simulink model "UnpackUDP"  (R2018b)
settings: configuration reference "Active" (kept outside this file)
undefined symbols (not defined in the file): tS, TUMHealthStatus
libraries: misc x5, etargetslib x5, simulink x2
settings Model: DataDictionary=UnpackUDP.sldd  sg_rtwmakecfg_data=_sg_IO821__sglibc_  Creator=lab1  LastModifiedBy=ge34qer

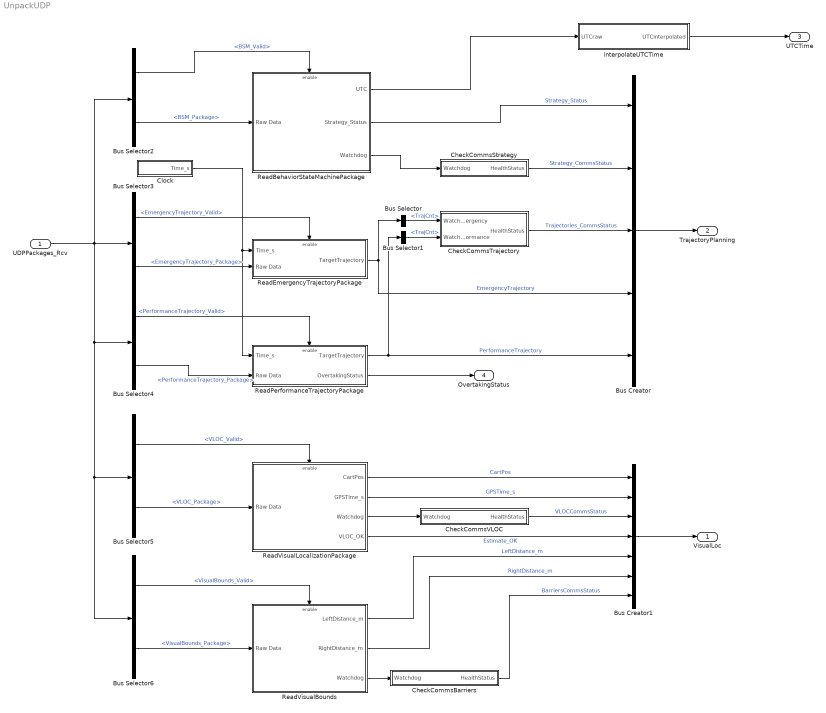
== system UnpackUDP ==
  UDPPackages_Rcv : Inport  OutDataTypeStr=Bus: UDPPackages_Rcv
  Bus Creator : BusCreator  Inputs=5
  Bus Creator1 : BusCreator  Inputs=7
  Bus Selector : BusSelector  OutputSignals=TrajCnt
  Bus Selector1 : BusSelector  OutputSignals=TrajCnt
  Bus Selector2 : BusSelector  OutputSignals=BSM_Valid,BSM_Package
  Bus Selector3 : BusSelector  OutputSignals=EmergencyTrajectory_Valid,EmergencyTrajectory_Package
  Bus Selector4 : BusSelector  OutputSignals=PerformanceTrajectory_Valid,PerformanceTrajectory_Package
  Bus Selector5 : BusSelector  OutputSignals=VLOC_Valid,VLOC_Package
  Bus Selector6 : BusSelector  OutputSignals=VisualBounds_Valid,VisualBounds_Package
  CheckCommsBarriers : Subsystem
  CheckCommsStrategy : Subsystem
  CheckCommsTrajectory : Subsystem
  CheckCommsVLOC : Subsystem
  Clock : Subsystem
  ReadBehaviorStateMachinePackage : Subsystem  Priority=1000
  ReadEmergencyTrajectoryPackage : Subsystem  Priority=1000
  ReadPerformanceTrajectoryPackage : Subsystem  Priority=1000
  ReadVisualBounds : Subsystem  Priority=1000
  ReadVisualLocalizationPackage : Subsystem  Priority=1000
  interpolateUTCTime : Subsystem
  VisualLoc : Outport  OutDataTypeStr=Bus: VisualLoc  BusOutputAsStruct=on
  TrajectoryPlanning : Outport  Port=2  OutDataTypeStr=Bus: TrajectoryPlanning  BusOutputAsStruct=on
  UTCTime : Outport  Port=3
  OvertakingStatus : Outport  Port=4  OutDataTypeStr=uint8
  wires:
  Bus Creator/1 -> TrajectoryPlanning/1
  ReadPerformanceTrajectoryPackage/1(TargetTrajectory) -> Bus Selector1/1, Bus Creator/5  "PerformanceTrajectory"
  ReadBehaviorStateMachinePackage/2(Strategy_Status) -> Bus Creator/1  "Strategy_Status"
  ReadBehaviorStateMachinePackage/3(Watchdog) -> CheckCommsStrategy/1(Watchdog)
  Bus Creator1/1 -> VisualLoc/1
  ReadVisualLocalizationPackage/2(GPSTime_s) -> Bus Creator1/2  "GPSTime_s"
  ReadVisualLocalizationPackage/1(CartPos) -> Bus Creator1/1  "CartPos"
  CheckCommsStrategy/1(HealthStatus) -> Bus Creator/2  "Strategy_CommsStatus"
  CheckCommsTrajectory/1(HealthStatus) -> Bus Creator/3  "Trajectories_CommsStatus"
  ReadEmergencyTrajectoryPackage/1(TargetTrajectory) -> Bus Creator/4, Bus Selector/1  "EmergencyTrajectory"
  Bus Selector/1 -> CheckCommsTrajectory/1(WatchdogEmergency)  "<TrajCnt>"
  Bus Selector1/1 -> CheckCommsTrajectory/2(WatchdogPerformance)  "<TrajCnt>"
  CheckCommsVLOC/1(HealthStatus) -> Bus Creator1/3  "VLOCCommsStatus"
  ReadVisualLocalizationPackage/4(VLOC_OK) -> Bus Creator1/4  "Estimate_OK"
  Clock/1(Time_s) -> ReadPerformanceTrajectoryPackage/1(Time_s), ReadEmergencyTrajectoryPackage/1(Time_s)
  UDPPackages_Rcv/1 -> Bus Selector2/1, Bus Selector6/1, Bus Selector5/1, Bus Selector4/1, Bus Selector3/1
  Bus Selector2/1 -> ReadBehaviorStateMachinePackage/Enable  "<BSM_Valid>"
  Bus Selector2/2 -> ReadBehaviorStateMachinePackage/1(Raw Data)  "<BSM_Package>"
  Bus Selector3/1 -> ReadEmergencyTrajectoryPackage/Enable  "<EmergencyTrajectory_Valid>"
  Bus Selector3/2 -> ReadEmergencyTrajectoryPackage/2(Raw Data)  "<EmergencyTrajectory_Package>"
  Bus Selector4/2 -> ReadPerformanceTrajectoryPackage/2(Raw Data)  "<PerformanceTrajectory_Package>"
  Bus Selector4/1 -> ReadPerformanceTrajectoryPackage/Enable  "<PerformanceTrajectory_Valid>"
  Bus Selector5/2 -> ReadVisualLocalizationPackage/1(Raw Data)  "<VLOC_Package>"
  Bus Selector5/1 -> ReadVisualLocalizationPackage/Enable  "<VLOC_Valid>"
  ReadVisualLocalizationPackage/3(Watchdog) -> CheckCommsVLOC/1(Watchdog)
  Bus Selector6/2 -> ReadVisualBounds/1(Raw Data)  "<VisualBounds_Package>"
  Bus Selector6/1 -> ReadVisualBounds/Enable  "<VisualBounds_Valid>"
  ReadVisualBounds/3(Watchdog) -> CheckCommsBarriers/1(Watchdog)
  ReadVisualBounds/1(LeftDistance_m) -> Bus Creator1/5  "LeftDistance_m"
  ReadVisualBounds/2(RightDistance_m) -> Bus Creator1/6  "RightDistance_m"
  CheckCommsBarriers/1(HealthStatus) -> Bus Creator1/7  "BarriersCommsStatus"
  interpolateUTCTime/1(UTCinterpolated) -> UTCTime/1
  ReadBehaviorStateMachinePackage/1(UTC) -> interpolateUTCTime/1(UTCraw)
  ReadPerformanceTrajectoryPackage/2(OvertakingStatus) -> OvertakingStatus/1

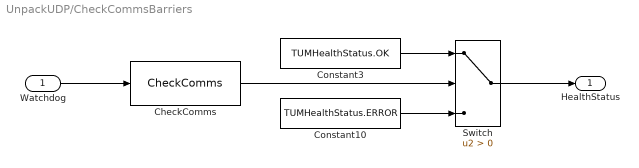
== system UnpackUDP/CheckCommsBarriers ==
  Watchdog : Inport
  CheckComms : misc/CheckComms  timeout_s=tPX2CommsTimeout  tS=tS
  Constant10 : Constant  Value=TUMHealthStatus.ERROR  OutDataTypeStr=Enum: TUMHealthStatus
  Constant3 : Constant  Value=TUMHealthStatus.OK  OutDataTypeStr=Enum: TUMHealthStatus
  Switch : Switch  Criteria=u2 > Threshold
  HealthStatus : Outport
  wires:
  Constant10/1 -> Switch/3
  CheckComms/1 -> Switch/2
  Constant3/1 -> Switch/1
  Switch/1 -> HealthStatus/1
  Watchdog/1 -> CheckComms/1

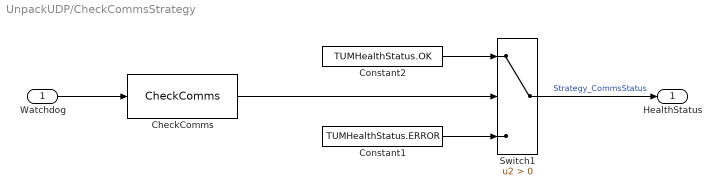
== system UnpackUDP/CheckCommsStrategy ==
  Watchdog : Inport
  CheckComms : misc/CheckComms  timeout_s=tPX2CommsTimeout  tS=tS
  Constant1 : Constant  Value=TUMHealthStatus.ERROR  OutDataTypeStr=Enum: TUMHealthStatus
  Constant2 : Constant  Value=TUMHealthStatus.OK  OutDataTypeStr=Enum: TUMHealthStatus
  Switch1 : Switch  Criteria=u2 > Threshold
  HealthStatus : Outport
  wires:
  CheckComms/1 -> Switch1/2
  Constant2/1 -> Switch1/1
  Switch1/1 -> HealthStatus/1  "Strategy_CommsStatus"
  Constant1/1 -> Switch1/3
  Watchdog/1 -> CheckComms/1

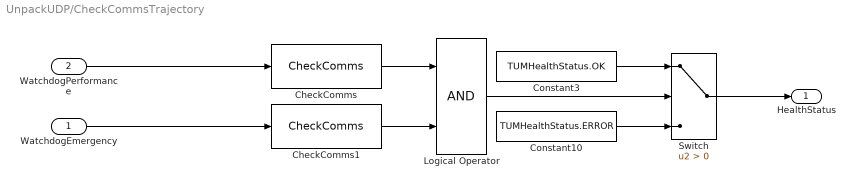
== system UnpackUDP/CheckCommsTrajectory ==
  WatchdogEmergency : Inport
  WatchdogPerformance : Inport  Port=2
  CheckComms : misc/CheckComms  timeout_s=tPX2CommsTimeout  tS=tS
  CheckComms1 : misc/CheckComms  timeout_s=tPX2CommsTimeout  tS=tS
  Constant10 : Constant  Value=TUMHealthStatus.ERROR  OutDataTypeStr=Enum: TUMHealthStatus
  Constant3 : Constant  Value=TUMHealthStatus.OK  OutDataTypeStr=Enum: TUMHealthStatus
  Logical Operator : Logic  AllPortsSameDT=off  OutDataTypeStr=boolean
  Switch : Switch  Criteria=u2 > Threshold
  HealthStatus : Outport
  wires:
  Constant10/1 -> Switch/3
  Logical Operator/1 -> Switch/2
  CheckComms/1 -> Logical Operator/1
  CheckComms1/1 -> Logical Operator/2
  Constant3/1 -> Switch/1
  Switch/1 -> HealthStatus/1
  WatchdogEmergency/1 -> CheckComms1/1
  WatchdogPerformance/1 -> CheckComms/1

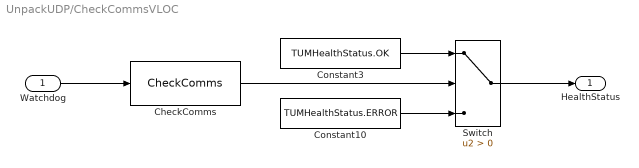
== system UnpackUDP/CheckCommsVLOC ==
  Watchdog : Inport
  CheckComms : misc/CheckComms  timeout_s=tPX2CommsTimeout  tS=tS
  Constant10 : Constant  Value=TUMHealthStatus.ERROR  OutDataTypeStr=Enum: TUMHealthStatus
  Constant3 : Constant  Value=TUMHealthStatus.OK  OutDataTypeStr=Enum: TUMHealthStatus
  Switch : Switch  Criteria=u2 > Threshold
  HealthStatus : Outport
  wires:
  Constant10/1 -> Switch/3
  CheckComms/1 -> Switch/2
  Constant3/1 -> Switch/1
  Switch/1 -> HealthStatus/1
  Watchdog/1 -> CheckComms/1

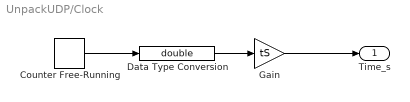
== system UnpackUDP/Clock ==
  Counter Free-Running : simulink/Sources/Counter Free-Running  NumBits=32  tsamp=tS
  Data Type Conversion : DataTypeConversion  OutDataTypeStr=double  SaturateOnIntegerOverflow=on
  Gain : Gain  Gain=tS
  Time_s : Outport
  wires:
  Counter Free-Running/1 -> Data Type Conversion/1
  Gain/1 -> Time_s/1
  Data Type Conversion/1 -> Gain/1

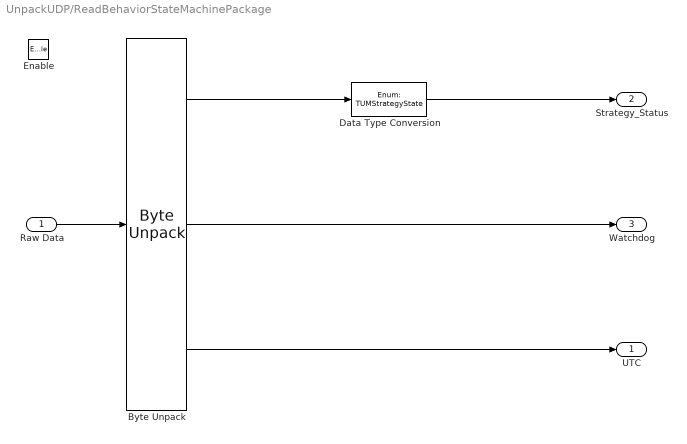
== system UnpackUDP/ReadBehaviorStateMachinePackage ==
  Raw Data : Inport
  Enable : EnablePort
  Byte Unpack : etargetslib/Byte Unpack  dimensions={[1], [1], [1]}  datatypes={'uint16', 'uint16', 'double'}  byteAlign=1
  Data Type Conversion : DataTypeConversion  OutDataTypeStr=Enum: TUMStrategyState  SaturateOnIntegerOverflow=on
  UTC : Outport
  Strategy_Status : Outport  Port=2  OutDataTypeStr=Enum: TUMStrategyState
  Watchdog : Outport  Port=3
  wires:
  Byte Unpack/1 -> Data Type Conversion/1
  Data Type Conversion/1 -> Strategy_Status/1
  Byte Unpack/2 -> Watchdog/1
  Raw Data/1 -> Byte Unpack/1
  Byte Unpack/3 -> UTC/1

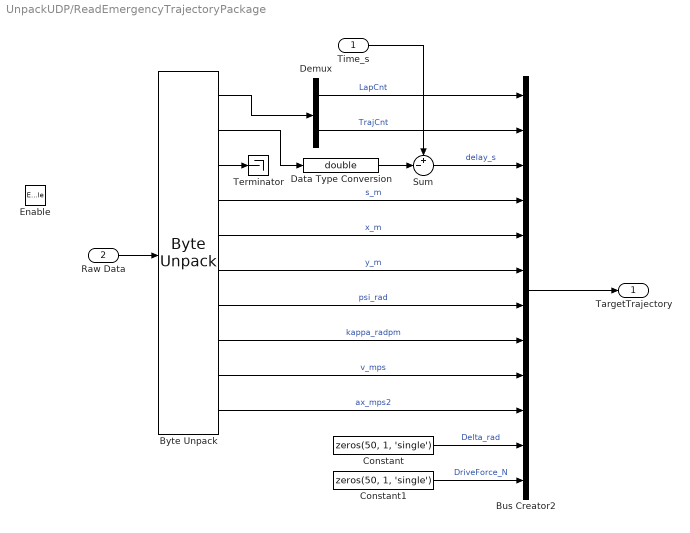
== system UnpackUDP/ReadEmergencyTrajectoryPackage ==
  Time_s : Inport
  Raw Data : Inport  Port=2
  Enable : EnablePort
  Bus Creator2 : BusCreator  Inputs=12  OutDataTypeStr=Bus: Trajectory
      settings: InheritFromInputs=off
  Byte Unpack : etargetslib/Byte Unpack  dimensions={[2], [1], [1], [50], [50], [50], [50], [50], [50],[50]}  datatypes={'uint32', 'single', 'uint8', 'single', 'single', 'single', 'single', 'single', 'single','single'}  byteAlign=1
  Constant : Constant  Value=zeros(50, 1, 'single')
  Constant1 : Constant  Value=zeros(50, 1, 'single')
  Data Type Conversion : DataTypeConversion  OutDataTypeStr=double  SaturateOnIntegerOverflow=on
  Demux : Demux  Outputs=2
  Sum : Sum  Inputs=+-|
  Terminator : Terminator
  TargetTrajectory : Outport  OutDataTypeStr=Bus: Trajectory
  wires:
  Byte Unpack/4 -> Bus Creator2/4  "s_m"
  Byte Unpack/5 -> Bus Creator2/5  "x_m"
  Byte Unpack/6 -> Bus Creator2/6  "y_m"
  Byte Unpack/7 -> Bus Creator2/7  "psi_rad"
  Byte Unpack/8 -> Bus Creator2/8  "kappa_radpm"
  Byte Unpack/9 -> Bus Creator2/9  "v_mps"
  Byte Unpack/10 -> Bus Creator2/10  "ax_mps2"
  Demux/1 -> Bus Creator2/1  "LapCnt"
  Demux/2 -> Bus Creator2/2  "TrajCnt"
  Bus Creator2/1 -> TargetTrajectory/1
  Byte Unpack/1 -> Demux/1
  Time_s/1 -> Sum/1
  Sum/1 -> Bus Creator2/3  "delay_s"
  Data Type Conversion/1 -> Sum/2
  Byte Unpack/2 -> Data Type Conversion/1
  Raw Data/1 -> Byte Unpack/1
  Constant/1 -> Bus Creator2/11  "Delta_rad"
  Constant1/1 -> Bus Creator2/12  "DriveForce_N"
  Byte Unpack/3 -> Terminator/1

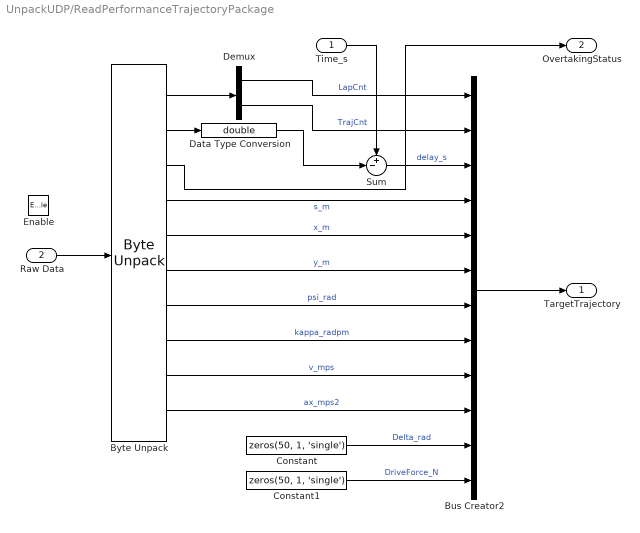
== system UnpackUDP/ReadPerformanceTrajectoryPackage ==
  Time_s : Inport
  Raw Data : Inport  Port=2
  Enable : EnablePort
  Bus Creator2 : BusCreator  Inputs=12  OutDataTypeStr=Bus: Trajectory
      settings: InheritFromInputs=off
  Byte Unpack : etargetslib/Byte Unpack  dimensions={[2], [1], [1], [50], [50], [50], [50], [50], [50],[50]}  datatypes={'uint32', 'single', 'uint8', 'single', 'single', 'single', 'single', 'single', 'single','single'}  byteAlign=1
  Constant : Constant  Value=zeros(50, 1, 'single')
  Constant1 : Constant  Value=zeros(50, 1, 'single')
  Data Type Conversion : DataTypeConversion  OutDataTypeStr=double  SaturateOnIntegerOverflow=on
  Demux : Demux  Outputs=2
  Sum : Sum  Inputs=+-|
  TargetTrajectory : Outport  OutDataTypeStr=Bus: Trajectory
  OvertakingStatus : Outport  Port=2
  wires:
  Byte Unpack/4 -> Bus Creator2/4  "s_m"
  Byte Unpack/5 -> Bus Creator2/5  "x_m"
  Byte Unpack/6 -> Bus Creator2/6  "y_m"
  Byte Unpack/7 -> Bus Creator2/7  "psi_rad"
  Byte Unpack/8 -> Bus Creator2/8  "kappa_radpm"
  Byte Unpack/9 -> Bus Creator2/9  "v_mps"
  Byte Unpack/10 -> Bus Creator2/10  "ax_mps2"
  Demux/1 -> Bus Creator2/1  "LapCnt"
  Demux/2 -> Bus Creator2/2  "TrajCnt"
  Bus Creator2/1 -> TargetTrajectory/1
  Time_s/1 -> Sum/1
  Data Type Conversion/1 -> Sum/2
  Sum/1 -> Bus Creator2/3  "delay_s"
  Byte Unpack/2 -> Data Type Conversion/1
  Raw Data/1 -> Byte Unpack/1
  Constant/1 -> Bus Creator2/11  "Delta_rad"
  Constant1/1 -> Bus Creator2/12  "DriveForce_N"
  Byte Unpack/1 -> Demux/1
  Byte Unpack/3 -> OvertakingStatus/1

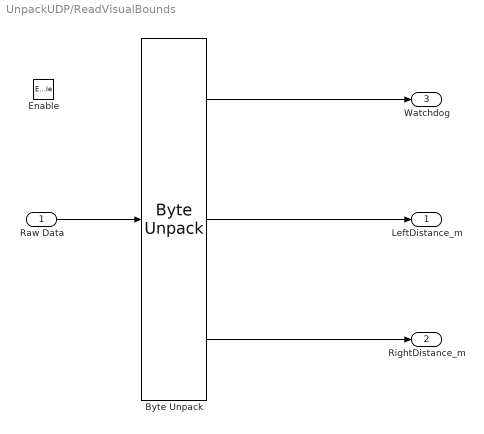
== system UnpackUDP/ReadVisualBounds ==
  Raw Data : Inport
  Enable : EnablePort
  Byte Unpack : etargetslib/Byte Unpack  dimensions={[1], [1], [1]}  datatypes={'double', 'double', 'double'}  byteAlign=1
  LeftDistance_m : Outport
  RightDistance_m : Outport  Port=2
  Watchdog : Outport  Port=3
  wires:
  Byte Unpack/1 -> Watchdog/1
  Raw Data/1 -> Byte Unpack/1
  Byte Unpack/2 -> LeftDistance_m/1
  Byte Unpack/3 -> RightDistance_m/1

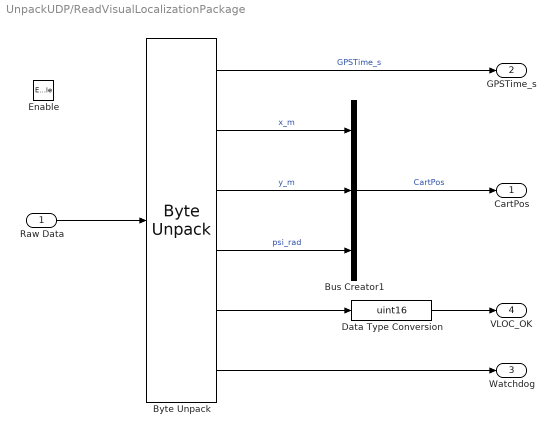
== system UnpackUDP/ReadVisualLocalizationPackage ==
  Raw Data : Inport
  Enable : EnablePort
  Bus Creator1 : BusCreator  Inputs=3
  Byte Unpack : etargetslib/Byte Unpack  dimensions={[1], [1], [1], [1], [1], [1]}  datatypes={'double', 'double', 'double', 'double', 'double', 'double'}  byteAlign=1
  Data Type Conversion : DataTypeConversion  OutDataTypeStr=uint16
  CartPos : Outport  OutDataTypeStr=Bus: CartPos
  GPSTime_s : Outport  Port=2
  Watchdog : Outport  Port=3
  VLOC_OK : Outport  Port=4
  wires:
  Bus Creator1/1 -> CartPos/1  "CartPos"
  Byte Unpack/3 -> Bus Creator1/2  "y_m"
  Byte Unpack/2 -> Bus Creator1/1  "x_m"
  Byte Unpack/1 -> GPSTime_s/1  "GPSTime_s"
  Byte Unpack/5 -> Data Type Conversion/1
  Data Type Conversion/1 -> VLOC_OK/1
  Raw Data/1 -> Byte Unpack/1
  Byte Unpack/4 -> Bus Creator1/3  "psi_rad"
  Byte Unpack/6 -> Watchdog/1

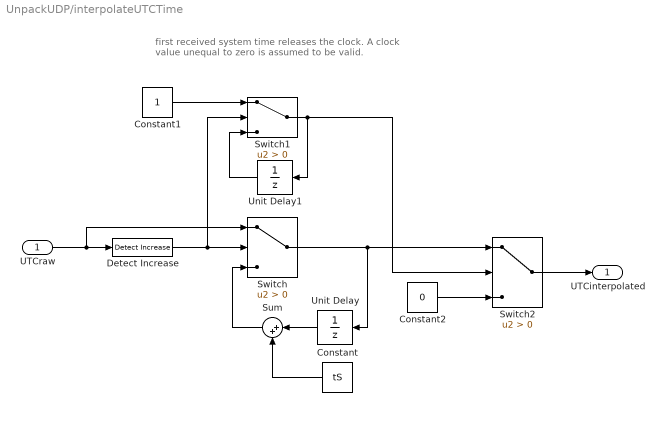
== system UnpackUDP/interpolateUTCTime ==
  note: first received system time releases the clock.
      | A clock value unequal to zero is assumed to be valid.
  UTCraw : Inport
  Constant : Constant  Value=tS
  Constant1 : Constant
  Constant2 : Constant  Value=0
  Detect Increase : simulink/Logic and Bit Operations/Detect Increase  vinit=0.0  OutDataTypeStr=boolean
  Sum : Sum  Inputs=|++
  Switch : Switch  Criteria=u2 > Threshold
  Switch1 : Switch  Criteria=u2 > Threshold
  Switch2 : Switch  Criteria=u2 > Threshold
  Unit Delay : UnitDelay  SampleTime=-1
  Unit Delay1 : UnitDelay  SampleTime=-1
  UTCinterpolated : Outport
  wires:
  UTCraw/1 -> Switch/1, Detect Increase/1
  Detect Increase/1 -> Switch1/2, Switch/2
  Sum/1 -> Switch/3
  Unit Delay/1 -> Sum/1
  Switch/1 -> Unit Delay/1, Switch2/1
  Constant/1 -> Sum/2
  Switch1/1 -> Unit Delay1/1, Switch2/2
  Unit Delay1/1 -> Switch1/3
  Constant1/1 -> Switch1/1
  Constant2/1 -> Switch2/3
  Switch2/1 -> UTCinterpolated/1
